simulink model "Product_Division"  (R2020a)
settings: Solver=VariableStepAuto  StartTime=0.0  StopTime=10.0  RelTol=1e-3
settings Model: Creator=royde  LastModifiedBy=royde

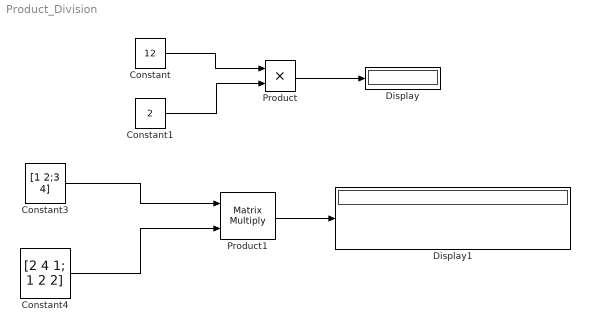
== system Product_Division ==
  Constant : Constant  Value=12
  Constant1 : Constant  Value=2
  Constant3 : Constant  Value=[1 2;3 4]
  Constant4 : Constant  Value=[2 4 1; 1 2 2]
  Display : Display
  Display1 : Display
  Product : Product
  Product1 : Product  Multiplication=Matrix(*)
  wires:
  Constant3/1 -> Product1/1
  Constant4/1 -> Product1/2
  Product1/1 -> Display1/1
  Product/1 -> Display/1
  Constant1/1 -> Product/2
  Constant/1 -> Product/1
